simulink model "Gewerk_2_v0_1"  (R2014a)
settings: Solver=ode45  StartTime=0.0  StopTime=17  RelTol=1e-3
libraries: dspswit3 x1
settings Model: Creator=ich  LastModifiedBy=ich

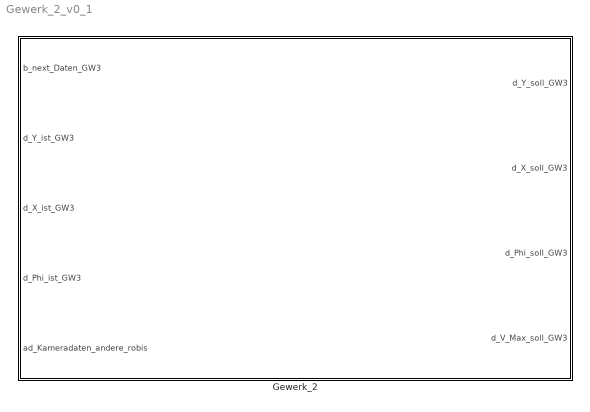
== system Gewerk_2_v0_1 ==
  Gewerk_2 : Subsystem

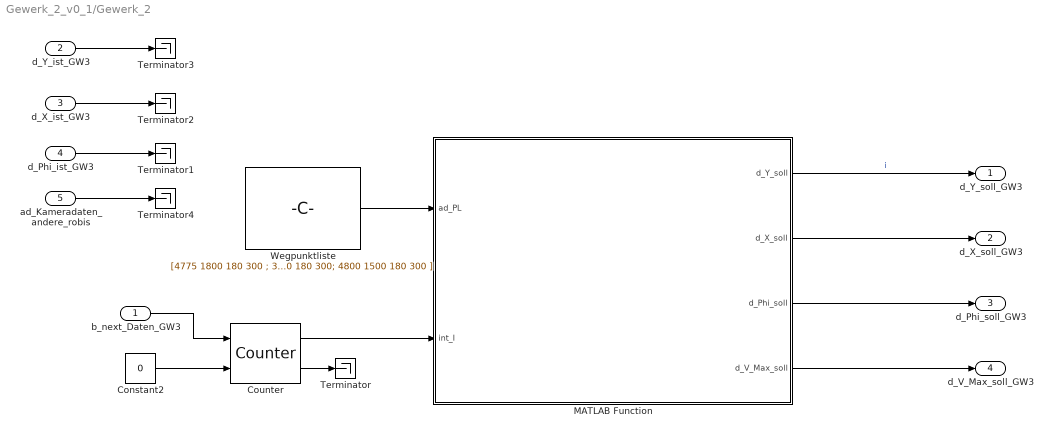
== system Gewerk_2_v0_1/Gewerk_2 ==
  b_next_Daten_GW3 : Inport  OutDataTypeStr=boolean
  d_Y_ist_GW3 : Inport  Port=2  OutDataTypeStr=boolean
  d_X_ist_GW3 : Inport  Port=3  OutDataTypeStr=boolean
  d_Phi_ist_GW3 : Inport  Port=4  OutDataTypeStr=boolean
  ad_Kameradaten_andere_robis : Inport  Port=5  OutDataTypeStr=boolean
  Constant2 : Constant  Value=0
  Counter : dspswit3/Counter  Direction=Up  CountEvent=Rising edge  CounterSize=User defined  MaxCount=16  InitialCount=0  Output=Count and Hit  HitValue=16  ResetInput=on  SamplesPerFrame=1  Ts=1  CntDtype=int32  HitDtype=Logical
  MATLAB Function : MATLAB Function  TreatAsAtomicUnit=on
  Terminator{,1..4} (5 alike) : Terminator
  Wegpunktliste : Constant  Value=[4775 1800 180 300 ; 3745 1800 180 300; 2540 2100 180 300; 2160 2100 180 300; 1678 1894 180 300; 1373 1846 180 300; 1155 1627 180 300; 1106 1321 180 300; 1246 1046 180 300; 1522 906 180 300; 1827 954 180 300; 2300 954 180 300; 2800 1500 180 300; 3300 1000 180 300; 3800 1500 180 300; 4300 1000 180 300; 4800 1500 180 300 ]  OutDataTypeStr=double
  d_Y_soll_GW3 : Outport  OutDataTypeStr=double
  d_X_soll_GW3 : Outport  Port=2  OutDataTypeStr=double
  d_Phi_soll_GW3 : Outport  Port=3  OutDataTypeStr=double
  d_V_Max_soll_GW3 : Outport  Port=4  OutDataTypeStr=double
  wires:
  d_Y_ist_GW3/1 -> Terminator3/1
  ad_Kameradaten_andere_robis/1 -> Terminator4/1
  d_Phi_ist_GW3/1 -> Terminator1/1
  d_X_ist_GW3/1 -> Terminator2/1
  Wegpunktliste/1 -> MATLAB Function/1(ad_PL)
  Counter/1 -> MATLAB Function/2(int_I)
  MATLAB Function/2(d_X_soll) -> d_X_soll_GW3/1
  b_next_Daten_GW3/1 -> Counter/1
  MATLAB Function/1(d_Y_soll) -> d_Y_soll_GW3/1  "i"
  MATLAB Function/4(d_V_Max_soll) -> d_V_Max_soll_GW3/1
  MATLAB Function/3(d_Phi_soll) -> d_Phi_soll_GW3/1
  Constant2/1 -> Counter/2
  Counter/2 -> Terminator/1

== matlab function Gewerk_2_v0_1/Gewerk_2/MATLAB Function ==
  data: ad_PL input; d_Y_soll output double; d_X_soll output double; d_Phi_soll output double; d_V_Max_soll output double; int_I input
function [d_Y_soll,d_X_soll,d_Phi_soll,d_V_Max_soll]= fcn(ad_PL,int_I)

int_I=int_I+1; %Offset, da Zeilenindex bei 1 beginnt

d_Y_soll= ad_PL(int_I,1);
d_X_soll= ad_PL(int_I,2);
d_Phi_soll= ad_PL(int_I,3);
d_V_Max_soll= ad_PL(int_I,4);
